simulink model "magic"  (R2019b)
settings: Solver=FixedStepAuto  StartTime=0.0  StopTime=18.06  FixedStep=0.005  RelTol=1e-3
libraries: dspfdesign x1
settings Model: Creator=USER  LastModifiedBy=USER

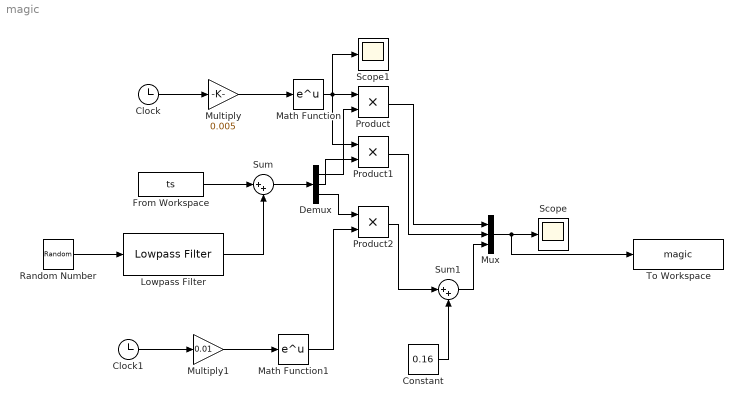
== system magic ==
  Clock : Clock
  Clock1 : Clock
  Constant : Constant  Value=0.16
  Demux : Demux  Outputs=3
  From Workspace : FromWorkspace  VariableName=ts  SampleTime=0
  Lowpass Filter : dspfdesign/Lowpass Filter  FilterType=FIR  DesignForMinimumOrder=on  FilterOrder=50  PassbandFrequency=8e2  StopbandFrequency=10e2  PassbandRipple=0.1  StopbandAttenuation=40  InheritSampleRate=off  SampleRate=44100  SimulateUsing=Interpreted execution  roundingMode=Floor  coeffsDataTypeStr=fixdt(1,16)
  Math Function : Math  SignedPower=off  SaturateOnIntegerOverflow=on
  Math Function1 : Math  SignedPower=off  SaturateOnIntegerOverflow=on
  Multiply : Gain  Gain=0.005
  Multiply1 : Gain  Gain=0.01
  Mux : Mux  Inputs=3
  Product : Product
  Product1 : Product
  Product2 : Product
  Random Number : RandomNumber  Variance=0.1  SampleTime=0.01
  Scope : Scope
  Scope1 : Scope
  Sum : Sum  Inputs=|++
  Sum1 : Sum  Inputs=|++
  To Workspace : ToWorkspace  VariableName=magic  SaveFormat=Timeseries  SampleTime=-1
  wires:
  From Workspace/1 -> Sum/1
  Random Number/1 -> Lowpass Filter/1
  Lowpass Filter/1 -> Sum/2
  Sum/1 -> Demux/1
  Clock/1 -> Multiply/1
  Multiply/1 -> Math Function/1
  Math Function/1 -> Product/1, Product1/1, Scope1/1
  Product/1 -> Mux/1
  Clock1/1 -> Multiply1/1
  Multiply1/1 -> Math Function1/1
  Demux/3 -> Product2/1
  Demux/2 -> Product1/2
  Demux/1 -> Product/2
  Math Function1/1 -> Product2/2
  Product1/1 -> Mux/2
  Mux/1 -> To Workspace/1, Scope/1
  Product2/1 -> Sum1/1
  Constant/1 -> Sum1/2
  Sum1/1 -> Mux/3
